simulink model "Function21"  (R2016b)
settings: Solver=VariableStepAuto  StartTime=0.0  StopTime=10.0  RelTol=1e-3
libraries: simulink x4
settings Model: Creator=viett  LastModifiedBy=viett

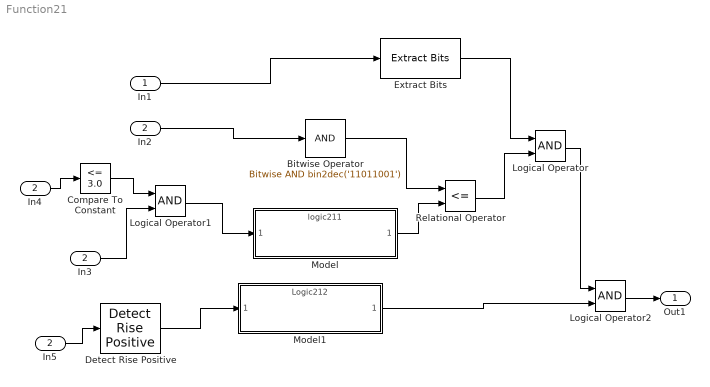
== system Function21 ==
  In1 : Inport
  In2 : Inport  Port=2
  Bitwise Operator : simulink/Logic and Bit Operations/Bitwise Operator  logicop=AND  UseBitMask=on  BitMask=bin2dec('11011001')  BitMaskRealWorld=Stored Integer
  Compare To Constant : simulink/Logic and Bit Operations/Compare To Constant  relop=<=  const=3.0  OutDataTypeStr=boolean
  Detect Rise Positive : simulink/Logic and Bit Operations/Detect Rise Positive  vinit=0  OutDataTypeStr=boolean
  Extract Bits : simulink/Logic and Bit Operations/Extract Bits  bitsToExtract=Upper half  numBits=8  bitIdxRange=[0 7]  outScalingMode=Preserve fixed-point scaling
  In3 : InportShadow  Port=2
  In4 : InportShadow  Port=2
  In5 : InportShadow  Port=2
  Logical Operator : Logic  AllPortsSameDT=off  OutDataTypeStr=boolean
  Logical Operator1 : Logic  AllPortsSameDT=off  OutDataTypeStr=boolean
  Logical Operator2 : Logic  AllPortsSameDT=off  OutDataTypeStr=boolean
  Model : ModelReference  ModelNameDialog=logic211.slx  SimulationMode=Normal  ModelReferenceVersion=1.9
  Model1 : ModelReference  ModelNameDialog=Logic212.slx  SimulationMode=Normal  ModelReferenceVersion=1.3
  Relational Operator : RelationalOperator  Operator=<=  OutDataTypeStr=boolean  RndMeth=Simplest
  Out1 : Outport
  wires:
  Logical Operator/1 -> Logical Operator2/1
  Extract Bits/1 -> Logical Operator/1
  Relational Operator/1 -> Logical Operator/2
  Model/1 -> Relational Operator/2
  Bitwise Operator/1 -> Relational Operator/1
  In1/1 -> Extract Bits/1
  Logical Operator1/1 -> Model/1
  In2/1 -> Bitwise Operator/1
  Compare To Constant/1 -> Logical Operator1/1
  In3/1 -> Logical Operator1/2
  In4/1 -> Compare To Constant/1
  Logical Operator2/1 -> Out1/1
  Model1/1 -> Logical Operator2/2
  Detect Rise Positive/1 -> Model1/1
  In5/1 -> Detect Rise Positive/1
